simulink model "QuarterCar_AFC_Replication"  (R2024b)
settings: Solver=ode4  StartTime=0.0  StopTime=20  FixedStep=0.001  RelTol=1e-3
settings Model: Creator=Galaba Vamsi  LastModifiedBy=Galaba Vamsi

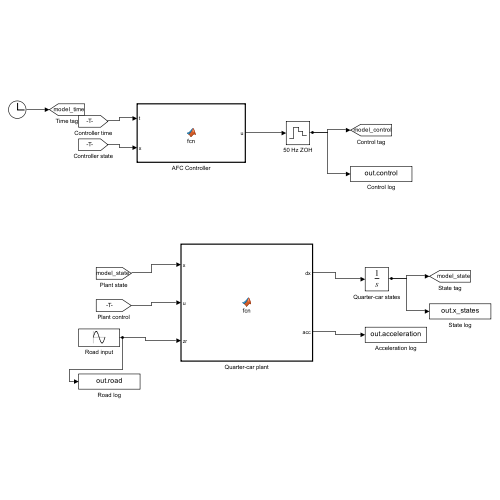
[thumbnail: Simulink's stored preview of the top-level diagram]
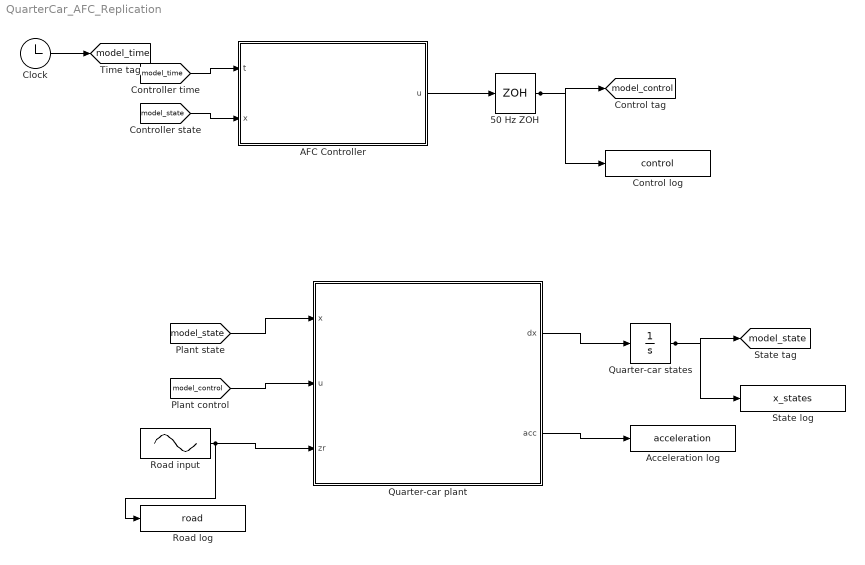
== system QuarterCar_AFC_Replication ==
  50 Hz ZOH : ZeroOrderHold  SampleTime=0.02
  AFC Controller : MATLAB Function  TreatAsAtomicUnit=on
  Acceleration log : ToWorkspace  VariableName=acceleration  SaveFormat=Timeseries  SampleTime=-1
  Clock : Clock
  Control log : ToWorkspace  VariableName=control  SaveFormat=Timeseries  SampleTime=-1
  Quarter-car plant : MATLAB Function  TreatAsAtomicUnit=on
  Quarter-car states : Integrator  InitialCondition=zeros(5,1)
  Road input : Sin  Amplitude=0.043  Frequency=3.173008580125691  SampleTime=0
  Road log : ToWorkspace  VariableName=road  SaveFormat=Timeseries  SampleTime=-1
  State log : ToWorkspace  VariableName=x_states  SaveFormat=Timeseries  SampleTime=-1
  tag scope: model_control=global, model_state=global, model_time=global
  wires:
  Clock/1 -> [model_time]
  [model_time] -> AFC Controller/1(t)
  [model_state] -> AFC Controller/2(x)
  AFC Controller/1(u) -> 50 Hz ZOH/1
  50 Hz ZOH/1 -> [model_control], Control log/1
  [model_state] -> Quarter-car plant/1(x)
  [model_control] -> Quarter-car plant/2(u)
  Road input/1 -> Quarter-car plant/3(zr), Road log/1
  Quarter-car plant/1(dx) -> Quarter-car states/1
  Quarter-car plant/2(acc) -> Acceleration log/1
  Quarter-car states/1 -> [model_state], State log/1

== matlab function QuarterCar_AFC_Replication/Quarter-car plant ==
  data: x input; u input; dx output; zr input; acc output
function [dx,acc] = fcn(x,u,zr)
ms=320; mu=40; ks=18000; ksn=0; bs=1000;
kt=200000; bt=0; area=0.000335; kappa=1e-06;
beta=1; cRel=0.05; bu=0.75; pressureLimit=10342500;
d=x(1)-x(3); v=x(2)-x(4);
Fs=ks*d+ksn*d^3; Fd=bs*v;
Ft=kt*(x(3)-zr); Fb=bt*x(4);
F=area*x(5)/kappa;
acc=(-Fd-Fs+F)/ms;
dx=zeros(5,1); dx(1)=x(2); dx(2)=acc; dx(3)=x(4);
dx(4)=(Fd+Fs-Ft-Fb-F)/mu;
dx(5)=-beta*x(5)-cRel*v+bu*u;
if x(5)>=kappa*pressureLimit && dx(5)>0, dx(5)=0; end
if x(5)<=-kappa*pressureLimit && dx(5)<0, dx(5)=0; end
end

== matlab function QuarterCar_AFC_Replication/AFC Controller ==
  data: t input; u output; x input
function u = fcn(t,x)
delta = 1; deltaBar = 1;
mu1 = (0.2-0.018)*exp(-3*t)+0.018;
mu2 = (110-90)*exp(-2*t)+90;
mu3 = (100-80)*exp(-2*t)+80;
z1 = min(max(x(1)/mu1,-delta+1e-8),deltaBar-1e-8);
e1 = 0.5*log((delta+z1)/(deltaBar-z1));
u1 = -25.5*e1;
z2 = min(max((x(2)-u1)/mu2,-delta+1e-8),deltaBar-1e-8);
e2 = 0.5*log((delta+z2)/(deltaBar-z2));
u2 = -12*e2;
z3 = min(max((x(5)-u2)/mu3,-delta+1e-8),deltaBar-1e-8);
e3 = 0.5*log((delta+z3)/(deltaBar-z3));
u = min(max(-216*e3,-5),5);
end
